simulink model "RCAM_OP_LONG_AP_SM_CL"  (R2022b)
settings: Solver=VariableStepAuto  StartTime=0.0  StopTime=10.0  RelTol=1e-3
undefined symbols (not defined in the file): H_nz, K_nzq
libraries: cstblocks x1
settings Model: Creator=bendr  LastModifiedBy=bendr

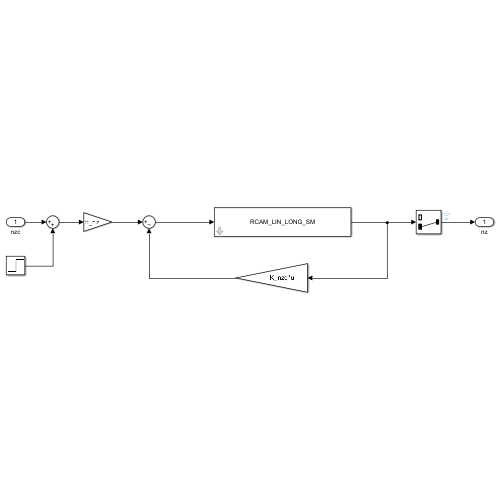
[thumbnail: Simulink's stored preview of the top-level diagram]
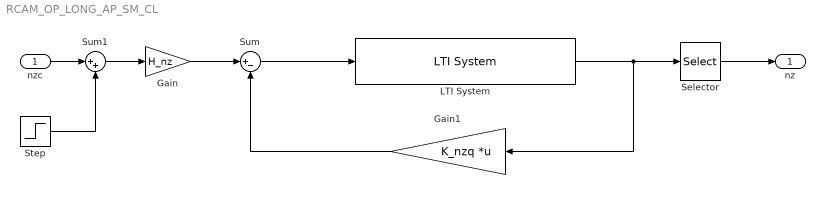
== system RCAM_OP_LONG_AP_SM_CL ==
  nzc : Inport
  Gain : Gain  Gain=H_nz
  Gain1 : Gain  Gain=K_nzq  Multiplication=Matrix(K*u)
  LTI System : cstblocks/LTI System  sys=RCAM_LIN_LONG_SM  IC=[]
  Selector : Selector  InputPortWidth=2  IndexOptions=Index vector (dialog)  Indices=2  OutputSizes=1
  Step : Step  SampleTime=0
  Sum : Sum  Inputs=|+-
  Sum1 : Sum  Inputs=|++
  nz : Outport
  wires:
  Gain/1 -> Sum/1
  Sum/1 -> LTI System/1
  Selector/1 -> nz/1
  LTI System/1 -> Gain1/1, Selector/1
  Gain1/1 -> Sum/2
  nzc/1 -> Sum1/1
  Sum1/1 -> Gain/1
  Step/1 -> Sum1/2
